simulink model "abc_to_alpha_beta"  (R2015a)
settings: Solver=ode3  StartTime=0.0  StopTime=10.0  FixedStep=0.001  RelTol=1e-3
settings Model: Creator=rblan  LastModifiedBy=rblan

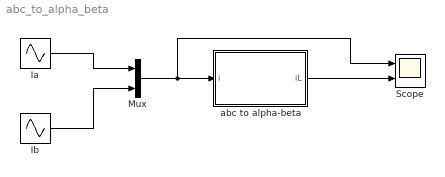
== system abc_to_alpha_beta ==
  Ia : Sin  Frequency=2*pi*50  SampleTime=0
  Ib : Sin  Frequency=2*pi*50  Phase=-2*pi/3  SampleTime=0
  Mux : Mux  Inputs=2
  Scope : Scope  NumInputPorts=2
      settings: ShowLegends=on  YMin=-5~-5  YMax=5~5
  abc to alpha-beta : Subsystem
  wires:
  Mux/1 -> Scope/1, abc to alpha-beta/1(i)
  abc to alpha-beta/1(iL) -> Scope/2
  Ia/1 -> Mux/1
  Ib/1 -> Mux/2

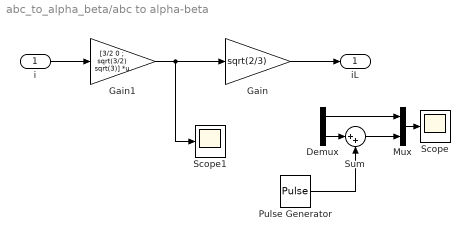
== system abc_to_alpha_beta/abc to alpha-beta ==
  i : Inport
  Demux : Demux  Outputs=2
  Gain : Gain  Gain=sqrt(2/3)
  Gain1 : Gain  Gain=[3/2 0 ; sqrt(3/2) sqrt(3)]  Multiplication=Matrix(K*u)
  Mux : Mux  Inputs=2
  Pulse Generator : DiscretePulseGenerator  PulseType=Time based  Period=1  PulseWidth=50
  Scope : Scope
      settings: ShowLegends=on
  Scope1 : Scope
      settings: ShowLegends=on  SaveName=ScopeData2
  Sum : Sum  Inputs=|++
  iL : Outport
  wires:
  i/1 -> Gain1/1
  Gain/1 -> iL/1
  Demux/2 -> Sum/1
  Pulse Generator/1 -> Sum/2
  Mux/1 -> Scope/1
  Sum/1 -> Mux/2
  Demux/1 -> Mux/1
  Gain1/1 -> Scope1/1, Gain/1
